simulink model "DCP_model"  (R2015b)
settings: Solver=ode3  StartTime=0.0  StopTime=inf  RelTol=1e-3
values from neighbouring files (symbols this model uses):
  numCars = 3    [Init_script.m]
undefined symbols (not defined in the file or in its folder): cars1, cars2, cars3, const, mat, param
libraries: CarMaker4SL x19, simulink x2
(part 2 of 2)

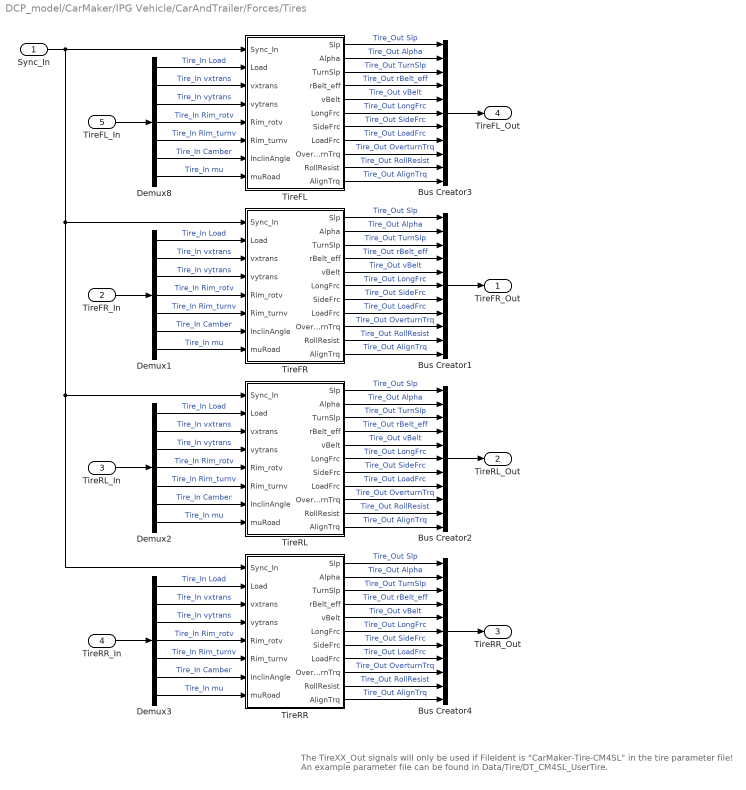
== system DCP_model/CarMaker/IPG Vehicle/CarAndTrailer/Forces/Tires ==
  note: The TireXX_Out signals will only be used if FileIdent is "CarMaker-Tire-CM4SL" in the tire parameter file!
      | An example parameter file can be found in Data/Tire/DT_CM4SL_UserTire.
  Sync_In : Inport
  TireFR_In : Inport  Port=2
  TireRL_In : Inport  Port=3
  TireRR_In : Inport  Port=4
  TireFL_In : Inport  Port=5
  Bus Creator{1..4} (4 alike) : BusCreator  Inputs=11
  Demux{1..3,8} (4 alike) : Demux  Outputs=7
  TireFL : Subsystem
  TireFR : Subsystem
  TireRL : Subsystem
  TireRR : Subsystem
  TireFR_Out : Outport
  TireRL_Out : Outport  Port=2
  TireRR_Out : Outport  Port=3
  TireFL_Out : Outport  Port=4
  wires:
  Sync_In/1 -> TireRR/1(Sync_In), TireRL/1(Sync_In), TireFR/1(Sync_In), TireFL/1(Sync_In)
  Bus Creator4/1 -> TireRR_Out/1
  Bus Creator2/1 -> TireRL_Out/1
  Bus Creator1/1 -> TireFR_Out/1
  Demux3/5 -> TireRR/6(Rim_turnv)  "Tire_In Rim_turnv"
  Demux3/4 -> TireRR/5(Rim_rotv)  "Tire_In Rim_rotv"
  Demux3/1 -> TireRR/2(Load)  "Tire_In Load"
  Demux3/7 -> TireRR/8(muRoad)  "Tire_In mu"
  Demux3/6 -> TireRR/7(InclinAngle)  "Tire_In Camber"
  Demux3/2 -> TireRR/3(vxtrans)  "Tire_In vxtrans"
  Demux3/3 -> TireRR/4(vytrans)  "Tire_In vytrans"
  TireRR/11(AlignTrq) -> Bus Creator4/11  "Tire_Out AlignTrq"
  TireRR/10(RollResist) -> Bus Creator4/10  "Tire_Out RollResist"
  TireRR/9(OverturnTrq) -> Bus Creator4/9  "Tire_Out OverturnTrq"
  TireRR/8(LoadFrc) -> Bus Creator4/8  "Tire_Out LoadFrc"
  TireRR/7(SideFrc) -> Bus Creator4/7  "Tire_Out SideFrc"
  TireRR/6(LongFrc) -> Bus Creator4/6  "Tire_Out LongFrc"
  TireRR/5(vBelt) -> Bus Creator4/5  "Tire_Out vBelt"
  TireRR/4(rBelt_eff) -> Bus Creator4/4  "Tire_Out rBelt_eff"
  TireRR/3(TurnSlp) -> Bus Creator4/3  "Tire_Out TurnSlp"
  TireRR/1(Slp) -> Bus Creator4/1  "Tire_Out Slp"
  TireRR/2(Alpha) -> Bus Creator4/2  "Tire_Out Alpha"
  Demux2/5 -> TireRL/6(Rim_turnv)  "Tire_In Rim_turnv"
  Demux2/4 -> TireRL/5(Rim_rotv)  "Tire_In Rim_rotv"
  Demux2/1 -> TireRL/2(Load)  "Tire_In Load"
  Demux2/7 -> TireRL/8(muRoad)  "Tire_In mu"
  Demux2/6 -> TireRL/7(InclinAngle)  "Tire_In Camber"
  Demux2/2 -> TireRL/3(vxtrans)  "Tire_In vxtrans"
  Demux2/3 -> TireRL/4(vytrans)  "Tire_In vytrans"
  TireRL/11(AlignTrq) -> Bus Creator2/11  "Tire_Out AlignTrq"
  TireRL/10(RollResist) -> Bus Creator2/10  "Tire_Out RollResist"
  TireRL/9(OverturnTrq) -> Bus Creator2/9  "Tire_Out OverturnTrq"
  TireRL/8(LoadFrc) -> Bus Creator2/8  "Tire_Out LoadFrc"
  TireRL/7(SideFrc) -> Bus Creator2/7  "Tire_Out SideFrc"
  TireRL/6(LongFrc) -> Bus Creator2/6  "Tire_Out LongFrc"
  TireRL/5(vBelt) -> Bus Creator2/5  "Tire_Out vBelt"
  TireRL/4(rBelt_eff) -> Bus Creator2/4  "Tire_Out rBelt_eff"
  TireRL/3(TurnSlp) -> Bus Creator2/3  "Tire_Out TurnSlp"
  TireRL/1(Slp) -> Bus Creator2/1  "Tire_Out Slp"
  TireRL/2(Alpha) -> Bus Creator2/2  "Tire_Out Alpha"
  Demux1/5 -> TireFR/6(Rim_turnv)  "Tire_In Rim_turnv"
  Demux1/4 -> TireFR/5(Rim_rotv)  "Tire_In Rim_rotv"
  Demux1/1 -> TireFR/2(Load)  "Tire_In Load"
  Demux1/7 -> TireFR/8(muRoad)  "Tire_In mu"
  Demux1/6 -> TireFR/7(InclinAngle)  "Tire_In Camber"
  Demux1/2 -> TireFR/3(vxtrans)  "Tire_In vxtrans"
  Demux1/3 -> TireFR/4(vytrans)  "Tire_In vytrans"
  TireFR/11(AlignTrq) -> Bus Creator1/11  "Tire_Out AlignTrq"
  TireFR/10(RollResist) -> Bus Creator1/10  "Tire_Out RollResist"
  TireFR/9(OverturnTrq) -> Bus Creator1/9  "Tire_Out OverturnTrq"
  TireFR/8(LoadFrc) -> Bus Creator1/8  "Tire_Out LoadFrc"
  TireFR/7(SideFrc) -> Bus Creator1/7  "Tire_Out SideFrc"
  TireFR/6(LongFrc) -> Bus Creator1/6  "Tire_Out LongFrc"
  TireFR/5(vBelt) -> Bus Creator1/5  "Tire_Out vBelt"
  TireFR/4(rBelt_eff) -> Bus Creator1/4  "Tire_Out rBelt_eff"
  TireFR/3(TurnSlp) -> Bus Creator1/3  "Tire_Out TurnSlp"
  TireFR/1(Slp) -> Bus Creator1/1  "Tire_Out Slp"
  TireFR/2(Alpha) -> Bus Creator1/2  "Tire_Out Alpha"
  Demux8/5 -> TireFL/6(Rim_turnv)  "Tire_In Rim_turnv"
  Demux8/4 -> TireFL/5(Rim_rotv)  "Tire_In Rim_rotv"
  TireFL_In/1 -> Demux8/1
  Demux8/1 -> TireFL/2(Load)  "Tire_In Load"
  Demux8/7 -> TireFL/8(muRoad)  "Tire_In mu"
  Demux8/6 -> TireFL/7(InclinAngle)  "Tire_In Camber"
  Demux8/2 -> TireFL/3(vxtrans)  "Tire_In vxtrans"
  Demux8/3 -> TireFL/4(vytrans)  "Tire_In vytrans"
  TireFL/11(AlignTrq) -> Bus Creator3/11  "Tire_Out AlignTrq"
  TireFL/10(RollResist) -> Bus Creator3/10  "Tire_Out RollResist"
  TireFL/9(OverturnTrq) -> Bus Creator3/9  "Tire_Out OverturnTrq"
  TireFL/8(LoadFrc) -> Bus Creator3/8  "Tire_Out LoadFrc"
  TireFL/7(SideFrc) -> Bus Creator3/7  "Tire_Out SideFrc"
  TireFL/6(LongFrc) -> Bus Creator3/6  "Tire_Out LongFrc"
  TireFL/5(vBelt) -> Bus Creator3/5  "Tire_Out vBelt"
  TireFL/4(rBelt_eff) -> Bus Creator3/4  "Tire_Out rBelt_eff"
  TireFL/3(TurnSlp) -> Bus Creator3/3  "Tire_Out TurnSlp"
  TireFL/1(Slp) -> Bus Creator3/1  "Tire_Out Slp"
  TireFL/2(Alpha) -> Bus Creator3/2  "Tire_Out Alpha"
  Bus Creator3/1 -> TireFL_Out/1
  TireFR_In/1 -> Demux1/1
  TireRL_In/1 -> Demux2/1
  TireRR_In/1 -> Demux3/1

== system DCP_model/CarMaker/IPG Vehicle/CarAndTrailer/Forces/Vehicle Forces ==
  Sync_In : Inport
  Bus Creator1 : BusCreator  Inputs=12
  Bus Creator5 : BusCreator  Inputs=13
  Bus Creator8 : BusCreator  Inputs=16
  Demux : Demux  Outputs=16
  Demux1 : Demux  Outputs=12
  Demux5 : Demux  Outputs=13
  Forces : S-Function  FunctionName=CM_Sfun  Parameters='Forces'  SFunctionDeploymentMode=off  EnableBusSupport=off
  Sync_Out : Outport
  Car.Virtual : Outport  Port=2
  Car.Aero : Outport  Port=3
  Car.Load : Outport  Port=4
  wires:
  Demux/16 -> Bus Creator8/16  "Car Load_3 tz"
  Demux/15 -> Bus Creator8/15  "Car Load_3 ty"
  Demux/14 -> Bus Creator8/14  "Car Load_3 tx"
  Demux/13 -> Bus Creator8/13  "Car Load_3 mass"
  Demux1/12 -> Bus Creator1/12  "Car Virtual Trq_0 z"
  Demux1/11 -> Bus Creator1/11  "Car Virtual Trq_0 y"
  Demux1/10 -> Bus Creator1/10  "Car Virtual Trq_0 x"
  Demux1/9 -> Bus Creator1/9  "Car Virtual Trq_1 z"
  Demux1/8 -> Bus Creator1/8  "Car Virtual Trq_1 y"
  Demux1/7 -> Bus Creator1/7  "Car Virtual Trq_1 x"
  Demux1/6 -> Bus Creator1/6  "Car Virtual Frc_0 z"
  Demux1/5 -> Bus Creator1/5  "Car Virtual Frc_0 y"
  Demux1/4 -> Bus Creator1/4  "Car Virtual Frc_0 x"
  Sync_In/1 -> Forces/1
  Forces/1 -> Sync_Out/1
  Bus Creator5/1 -> Car.Aero/1
  Demux1/1 -> Bus Creator1/1  "Car Virtual Frc_1 x"
  Demux1/2 -> Bus Creator1/2  "Car Virtual Frc_1 y"
  Demux1/3 -> Bus Creator1/3  "Car Virtual Frc_1 z"
  Forces/3 -> Demux5/1
  Forces/2 -> Demux1/1
  Bus Creator1/1 -> Car.Virtual/1
  Bus Creator8/1 -> Car.Load/1
  Demux/1 -> Bus Creator8/1  "Car Load_0 mass"
  Demux/2 -> Bus Creator8/2  "Car Load_0 tx"
  Demux/3 -> Bus Creator8/3  "Car Load_0 ty"
  Demux/4 -> Bus Creator8/4  "Car Load_0 tz"
  Demux/5 -> Bus Creator8/5  "Car Load_1 mass"
  Demux/6 -> Bus Creator8/6  "Car Load_1 tx"
  Demux/7 -> Bus Creator8/7  "Car Load_1 ty"
  Demux/8 -> Bus Creator8/8  "Car Load_1 tz"
  Demux/9 -> Bus Creator8/9  "Car Load_2 mass"
  Demux/10 -> Bus Creator8/10  "Car Load_2 tx"
  Demux/11 -> Bus Creator8/11  "Car Load_2 ty"
  Demux/12 -> Bus Creator8/12  "Car Load_2 tz"
  Forces/4 -> Demux/1
  Demux5/11 -> Bus Creator5/11  "car Aero Trq_1 x"
  Demux5/12 -> Bus Creator5/12  "car Aero Trq_1 y"
  Demux5/13 -> Bus Creator5/13  "car Aero Trq_1 z"
  Demux5/10 -> Bus Creator5/10  "car Aero Frc_1 z"
  Demux5/9 -> Bus Creator5/9  "car Aero Frc_1 y"
  Demux5/8 -> Bus Creator5/8  "car Aero Frc_1 x"
  Demux5/1 -> Bus Creator5/1  "Vehicle sRoadAero"
  Demux5/2 -> Bus Creator5/2  "Vehicle Wind_vel_0 x"
  Demux5/3 -> Bus Creator5/3  "Vehicle Wind_vel_0 y"
  Demux5/4 -> Bus Creator5/4  "Vehicle Wind_vel_0 z"
  Demux5/5 -> Bus Creator5/5  "car Aero vRes_1 x"
  Demux5/6 -> Bus Creator5/6  "car Aero vRes_1 y"
  Demux5/7 -> Bus Creator5/7  "car Aero vRes_1 z"

== system DCP_model/CarMaker/IPG Vehicle/CarAndTrailer/Trailer/CreateBus Car.Hitch.FrcTrq ==
  In1 : Inport
  Bus Creator7 : BusCreator  Inputs=6
  Demux7 : Demux  Outputs=6
  Car.Hitch.FrcTrq : Outport
  wires:
  In1/1 -> Demux7/1
  Bus Creator7/1 -> Car.Hitch.FrcTrq/1
  Demux7/6 -> Bus Creator7/6  "Car Hitch Trq2Car z"
  Demux7/5 -> Bus Creator7/5  "Car Hitch Trq2Car y"
  Demux7/4 -> Bus Creator7/4  "Car Hitch Trq2Car x"
  Demux7/3 -> Bus Creator7/3  "Car Hitch Frc2Car z"
  Demux7/2 -> Bus Creator7/2  "Car Hitch Frc2Car y"
  Demux7/1 -> Bus Creator7/1  "Car Hitch Frc2Car x"

== system DCP_model/CarMaker/IPG Vehicle/CarAndTrailer/Trailer/CreateBus Vhcl.Motion ==
  In1 : Inport
  Demux1 : Demux  Outputs=16
  Mux1 : Mux  Inputs=16
  Out1 : Outport
  wires:
  Demux1/1 -> Mux1/1  "Vhcl v"
  Demux1/2 -> Mux1/2  "Vhcl Distance"
  Demux1/3 -> Mux1/3  "Vhcl sRoad"
  Demux1/4 -> Mux1/4  "Vhcl sRoadAero"
  Demux1/5 -> Mux1/5  "Vhcl Hitch_Pos x"
  Demux1/6 -> Mux1/6  "Vhcl Hitch_Pos y"
  Demux1/7 -> Mux1/7  "Vhcl Hitch_Pos z"
  Demux1/8 -> Mux1/8  "Vhcl Roll"
  Demux1/9 -> Mux1/9  "Vhcl RollVel"
  Demux1/10 -> Mux1/10  "Vhcl RollAcc"
  Demux1/11 -> Mux1/11  "Vhcl Pitch"
  Demux1/12 -> Mux1/12  "Vhcl PitchVel"
  Demux1/13 -> Mux1/13  "Vhcl PitchAcc"
  Demux1/14 -> Mux1/14  "Vhcl Yaw"
  Demux1/15 -> Mux1/15  "Vhcl YawRate"
  Demux1/16 -> Mux1/16  "Vhcl YawAcc"
  In1/1 -> Demux1/1
  Mux1/1 -> Out1/1

== system DCP_model/CarMaker/IPG Vehicle/CarAndTrailer/Trailer/CreateBus Vhcl.PoI ==
  In1 : Inport
  Bus Creator3 : BusCreator  Inputs=18
  Demux3 : Demux  Outputs=18
  Out1 : Outport
  wires:
  Demux3/18 -> Bus Creator3/18  "Vhcl PoI_GCS Elev"
  Demux3/17 -> Bus Creator3/17  "Vhcl PoI_GCS Lat"
  Demux3/16 -> Bus Creator3/16  "Vhcl PoI_GCS Long"
  Demux3/15 -> Bus Creator3/15  "Vhcl PoI_Acc_1 z"
  Demux3/14 -> Bus Creator3/14  "Vhcl PoI_Acc_1 y"
  Demux3/13 -> Bus Creator3/13  "Vhcl PoI_Acc_1 x"
  Demux3/12 -> Bus Creator3/12  "Vhcl PoI_Vel_1 z"
  Demux3/11 -> Bus Creator3/11  "Vhcl PoI_Vel_1 y"
  Demux3/10 -> Bus Creator3/10  "Vhcl PoI_Vel_1 x"
  Demux3/9 -> Bus Creator3/9  "Vhcl PoI_Acc z"
  Demux3/8 -> Bus Creator3/8  "Vhcl PoI_Acc y"
  Demux3/7 -> Bus Creator3/7  "Vhcl PoI_Acc x"
  Demux3/6 -> Bus Creator3/6  "Vhcl PoI_Vel z"
  Demux3/5 -> Bus Creator3/5  "Vhcl PoI_Vel y"
  Demux3/4 -> Bus Creator3/4  "Vhcl PoI_Vel x"
  Demux3/3 -> Bus Creator3/3  "Vhcl PoI_Pos z"
  Demux3/2 -> Bus Creator3/2  "Vhcl PoI_Pos y"
  In1/1 -> Demux3/1
  Bus Creator3/1 -> Out1/1
  Demux3/1 -> Bus Creator3/1  "Vhcl PoI_Pos x"

== system DCP_model/CarMaker/IPG Vehicle/CarAndTrailer/Trailer/CreateBus Vhcl.Steering ==
  In1 : Inport
  Bus Creator3 : BusCreator  Inputs=4
  Demux : Demux
  Out1 : Outport
  wires:
  Bus Creator3/1 -> Out1/1
  Demux/1 -> Bus Creator3/1  "Vhcl Steering Ang"
  Demux/3 -> Bus Creator3/3  "Vhcl Steering AngAcc"
  Demux/2 -> Bus Creator3/2  "Vhcl Steering AngVel"
  Demux/4 -> Bus Creator3/4  "Vhcl Steering Trq"
  In1/1 -> Demux/1

== system DCP_model/CarMaker/IPG Vehicle/CarAndTrailer/Trailer/CreateBus Vhcl.Wheel.FL ==
  In1 : Inport
  Bus Creator3 : BusCreator  Inputs=14
  Demux3 : Demux  Outputs=14
  Out1 : Outport
  wires:
  Demux3/14 -> Bus Creator3/14  "Vhcl Wheel FL Trq_WhlBearing"
  Demux3/13 -> Bus Creator3/13  "Vhcl Wheel FL Trq_T2W"
  Demux3/12 -> Bus Creator3/12  "Vhcl Wheel FL SideSlip"
  Demux3/11 -> Bus Creator3/11  "Vhcl Wheel FL LongSlip"
  Demux3/10 -> Bus Creator3/10  "Vhcl Wheel FL vBelt"
  Demux3/9 -> Bus Creator3/9  "Vhcl Wheel FL Fz"
  Demux3/8 -> Bus Creator3/8  "Vhcl Wheel FL Fy"
  Demux3/7 -> Bus Creator3/7  "Vhcl Wheel FL Fx"
  Demux3/6 -> Bus Creator3/6  "Vhcl Wheel FL r_zxy z"
  Demux3/5 -> Bus Creator3/5  "Vhcl Wheel FL r_zxy y"
  Demux3/4 -> Bus Creator3/4  "Vhcl Wheel FL r_zxy x"
  Demux3/3 -> Bus Creator3/3  "Vhcl Wheel FL t z"
  Demux3/2 -> Bus Creator3/2  "Vhcl Wheel FL t y"
  In1/1 -> Demux3/1
  Bus Creator3/1 -> Out1/1
  Demux3/1 -> Bus Creator3/1  "Vhcl Wheel FL t x"

== system DCP_model/CarMaker/IPG Vehicle/CarAndTrailer/Trailer/CreateBus Vhcl.Wheel.FR ==
  In1 : Inport
  Bus Creator3 : BusCreator  Inputs=14
  Demux3 : Demux  Outputs=14
  Out1 : Outport
  wires:
  Demux3/14 -> Bus Creator3/14  "Vhcl Wheel FR Trq_WhlBearing"
  Demux3/13 -> Bus Creator3/13  "Vhcl Wheel FR Trq_T2W"
  Demux3/12 -> Bus Creator3/12  "Vhcl Wheel FR SideSlip"
  Demux3/11 -> Bus Creator3/11  "Vhcl Wheel FR LongSlip"
  Demux3/10 -> Bus Creator3/10  "Vhcl Wheel FR vBelt"
  Demux3/9 -> Bus Creator3/9  "Vhcl Wheel FR Fz"
  Demux3/8 -> Bus Creator3/8  "Vhcl Wheel FR Fy"
  Demux3/7 -> Bus Creator3/7  "Vhcl Wheel FR Fx"
  Demux3/6 -> Bus Creator3/6  "Vhcl Wheel FR r_zxy z"
  Demux3/5 -> Bus Creator3/5  "Vhcl Wheel FR r_zxy y"
  Demux3/4 -> Bus Creator3/4  "Vhcl Wheel FR r_zxy x"
  Demux3/3 -> Bus Creator3/3  "Vhcl Wheel FR t z"
  Demux3/2 -> Bus Creator3/2  "Vhcl Wheel FR t y"
  In1/1 -> Demux3/1
  Bus Creator3/1 -> Out1/1
  Demux3/1 -> Bus Creator3/1  "Vhcl Wheel FR t x"

== system DCP_model/CarMaker/IPG Vehicle/CarAndTrailer/Trailer/CreateBus Vhcl.Wheel.RL ==
  In1 : Inport
  Bus Creator3 : BusCreator  Inputs=14
  Demux3 : Demux  Outputs=14
  Out1 : Outport
  wires:
  Demux3/14 -> Bus Creator3/14  "Vhcl Wheel RL Trq_WhlBearing"
  Demux3/13 -> Bus Creator3/13  "Vhcl Wheel RL Trq_T2W"
  Demux3/12 -> Bus Creator3/12  "Vhcl Wheel RL SideSlip"
  Demux3/11 -> Bus Creator3/11  "Vhcl Wheel RL LongSlip"
  Demux3/10 -> Bus Creator3/10  "Vhcl Wheel RL vBelt"
  Demux3/9 -> Bus Creator3/9  "Vhcl Wheel RL Fz"
  Demux3/8 -> Bus Creator3/8  "Vhcl Wheel RL Fy"
  Demux3/7 -> Bus Creator3/7  "Vhcl Wheel RL Fx"
  Demux3/6 -> Bus Creator3/6  "Vhcl Wheel RL r_zxy z"
  Demux3/5 -> Bus Creator3/5  "Vhcl Wheel RL r_zxy y"
  Demux3/4 -> Bus Creator3/4  "Vhcl Wheel RL r_zxy x"
  Demux3/3 -> Bus Creator3/3  "Vhcl Wheel RL t z"
  Demux3/2 -> Bus Creator3/2  "Vhcl Wheel RL t y"
  In1/1 -> Demux3/1
  Bus Creator3/1 -> Out1/1
  Demux3/1 -> Bus Creator3/1  "Vhcl Wheel RL t x"

== system DCP_model/CarMaker/IPG Vehicle/CarAndTrailer/Trailer/CreateBus Vhcl.Wheel.RR ==
  In1 : Inport
  Bus Creator3 : BusCreator  Inputs=14
  Demux3 : Demux  Outputs=14
  Out1 : Outport
  wires:
  Demux3/14 -> Bus Creator3/14  "Vhcl Wheel RR Trq_WhlBearing"
  Demux3/13 -> Bus Creator3/13  "Vhcl Wheel RR Trq_T2W"
  Demux3/12 -> Bus Creator3/12  "Vhcl Wheel RR SideSlip"
  Demux3/11 -> Bus Creator3/11  "Vhcl Wheel RR LongSlip"
  Demux3/10 -> Bus Creator3/10  "Vhcl Wheel RR vBelt"
  Demux3/9 -> Bus Creator3/9  "Vhcl Wheel RR Fz"
  Demux3/8 -> Bus Creator3/8  "Vhcl Wheel RR Fy"
  Demux3/7 -> Bus Creator3/7  "Vhcl Wheel RR Fx"
  Demux3/6 -> Bus Creator3/6  "Vhcl Wheel RR r_zxy z"
  Demux3/5 -> Bus Creator3/5  "Vhcl Wheel RR r_zxy y"
  Demux3/4 -> Bus Creator3/4  "Vhcl Wheel RR r_zxy x"
  Demux3/3 -> Bus Creator3/3  "Vhcl Wheel RR t z"
  Demux3/2 -> Bus Creator3/2  "Vhcl Wheel RR t y"
  In1/1 -> Demux3/1
  Bus Creator3/1 -> Out1/1
  Demux3/1 -> Bus Creator3/1  "Vhcl Wheel RR t x"

== system DCP_model/CarMaker/VehicleControl/AccelCtrl1/PI-Controller/Integrator ==
  I-Part : Inport
  AxCtrl On : Inport  Port=2
  Init I-part : Inport  Port=3
  Add1 : Sum  SaturateOnIntegerOverflow=on  OutDataTypeStr=Inherit: Same as first input
  Memory : Memory
  Saturation : Saturate  UpperLimit=1  LowerLimit=-1
  Switch Ax Init I-Part : Switch  Threshold=1  SaturateOnIntegerOverflow=on
  "I-part tot " : Outport
  wires:
  Init I-part/1 -> Switch Ax Init I-Part/3
  Memory/1 -> Switch Ax Init I-Part/1
  AxCtrl On/1 -> Switch Ax Init I-Part/2
  I-Part/1 -> Add1/1
  Add1/1 -> "I-part tot "/1, Saturation/1
  Switch Ax Init I-Part/1 -> Add1/2
  Saturation/1 -> Memory/1

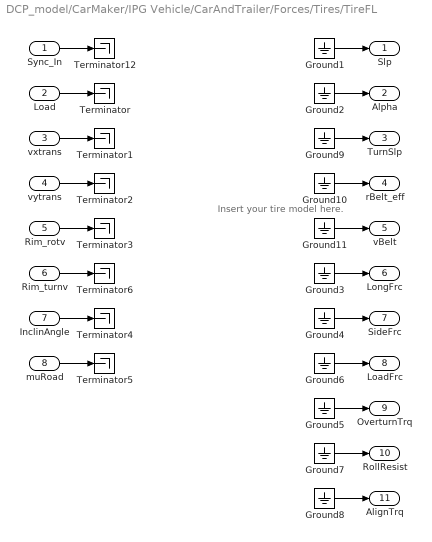
== system DCP_model/CarMaker/IPG Vehicle/CarAndTrailer/Forces/Tires/TireFL ==
  note: Insert your tire model here.
  Sync_In : Inport
  Load : Inport  Port=2
  vxtrans : Inport  Port=3
  vytrans : Inport  Port=4
  Rim_rotv : Inport  Port=5
  Rim_turnv : Inport  Port=6
  InclinAngle : Inport  Port=7
  muRoad : Inport  Port=8
  Ground{1..11} (11 alike) : Ground
  Terminator{,1..6,12} (8 alike) : Terminator
  Slp : Outport
  Alpha : Outport  Port=2
  TurnSlp : Outport  Port=3
  rBelt_eff : Outport  Port=4
  vBelt : Outport  Port=5
  LongFrc : Outport  Port=6
  SideFrc : Outport  Port=7
  LoadFrc : Outport  Port=8
  OverturnTrq : Outport  Port=9
  RollResist : Outport  Port=10
  AlignTrq : Outport  Port=11
  wires:
  Ground11/1 -> vBelt/1
  Ground10/1 -> rBelt_eff/1
  Ground9/1 -> TurnSlp/1
  Rim_turnv/1 -> Terminator6/1
  Sync_In/1 -> Terminator12/1
  Ground2/1 -> Alpha/1
  Ground3/1 -> LongFrc/1
  Ground4/1 -> SideFrc/1
  Ground5/1 -> OverturnTrq/1
  vxtrans/1 -> Terminator1/1
  vytrans/1 -> Terminator2/1
  Rim_rotv/1 -> Terminator3/1
  InclinAngle/1 -> Terminator4/1
  muRoad/1 -> Terminator5/1
  Load/1 -> Terminator/1
  Ground1/1 -> Slp/1
  Ground6/1 -> LoadFrc/1
  Ground7/1 -> RollResist/1
  Ground8/1 -> AlignTrq/1

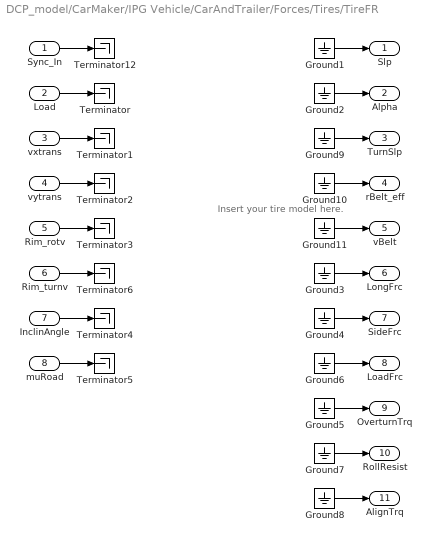
== system DCP_model/CarMaker/IPG Vehicle/CarAndTrailer/Forces/Tires/TireFR ==
  note: Insert your tire model here.
  Sync_In : Inport
  Load : Inport  Port=2
  vxtrans : Inport  Port=3
  vytrans : Inport  Port=4
  Rim_rotv : Inport  Port=5
  Rim_turnv : Inport  Port=6
  InclinAngle : Inport  Port=7
  muRoad : Inport  Port=8
  Ground{1..11} (11 alike) : Ground
  Terminator{,1..6,12} (8 alike) : Terminator
  Slp : Outport
  Alpha : Outport  Port=2
  TurnSlp : Outport  Port=3
  rBelt_eff : Outport  Port=4
  vBelt : Outport  Port=5
  LongFrc : Outport  Port=6
  SideFrc : Outport  Port=7
  LoadFrc : Outport  Port=8
  OverturnTrq : Outport  Port=9
  RollResist : Outport  Port=10
  AlignTrq : Outport  Port=11
  wires:
  Ground11/1 -> vBelt/1
  Ground10/1 -> rBelt_eff/1
  Ground9/1 -> TurnSlp/1
  Rim_turnv/1 -> Terminator6/1
  Sync_In/1 -> Terminator12/1
  Ground2/1 -> Alpha/1
  Ground3/1 -> LongFrc/1
  Ground4/1 -> SideFrc/1
  Ground5/1 -> OverturnTrq/1
  vxtrans/1 -> Terminator1/1
  vytrans/1 -> Terminator2/1
  Rim_rotv/1 -> Terminator3/1
  InclinAngle/1 -> Terminator4/1
  muRoad/1 -> Terminator5/1
  Load/1 -> Terminator/1
  Ground1/1 -> Slp/1
  Ground6/1 -> LoadFrc/1
  Ground7/1 -> RollResist/1
  Ground8/1 -> AlignTrq/1

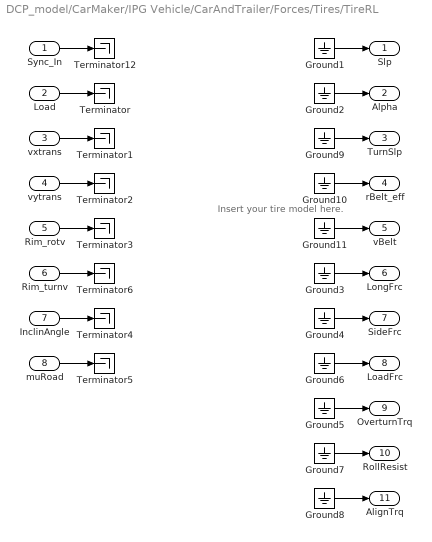
== system DCP_model/CarMaker/IPG Vehicle/CarAndTrailer/Forces/Tires/TireRL ==
  note: Insert your tire model here.
  Sync_In : Inport
  Load : Inport  Port=2
  vxtrans : Inport  Port=3
  vytrans : Inport  Port=4
  Rim_rotv : Inport  Port=5
  Rim_turnv : Inport  Port=6
  InclinAngle : Inport  Port=7
  muRoad : Inport  Port=8
  Ground{1..11} (11 alike) : Ground
  Terminator{,1..6,12} (8 alike) : Terminator
  Slp : Outport
  Alpha : Outport  Port=2
  TurnSlp : Outport  Port=3
  rBelt_eff : Outport  Port=4
  vBelt : Outport  Port=5
  LongFrc : Outport  Port=6
  SideFrc : Outport  Port=7
  LoadFrc : Outport  Port=8
  OverturnTrq : Outport  Port=9
  RollResist : Outport  Port=10
  AlignTrq : Outport  Port=11
  wires:
  Ground11/1 -> vBelt/1
  Ground10/1 -> rBelt_eff/1
  Ground9/1 -> TurnSlp/1
  Rim_turnv/1 -> Terminator6/1
  Sync_In/1 -> Terminator12/1
  Ground2/1 -> Alpha/1
  Ground3/1 -> LongFrc/1
  Ground4/1 -> SideFrc/1
  Ground5/1 -> OverturnTrq/1
  vxtrans/1 -> Terminator1/1
  vytrans/1 -> Terminator2/1
  Rim_rotv/1 -> Terminator3/1
  InclinAngle/1 -> Terminator4/1
  muRoad/1 -> Terminator5/1
  Load/1 -> Terminator/1
  Ground1/1 -> Slp/1
  Ground6/1 -> LoadFrc/1
  Ground7/1 -> RollResist/1
  Ground8/1 -> AlignTrq/1

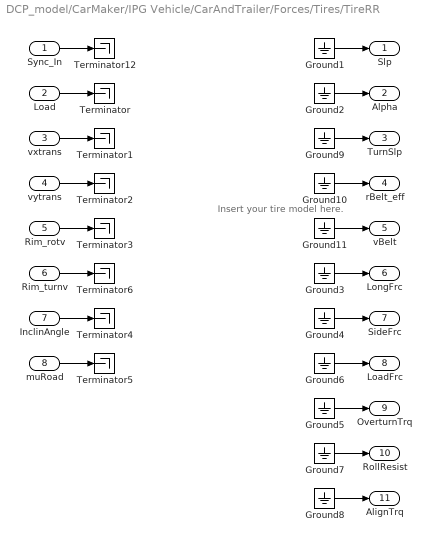
== system DCP_model/CarMaker/IPG Vehicle/CarAndTrailer/Forces/Tires/TireRR ==
  note: Insert your tire model here.
  Sync_In : Inport
  Load : Inport  Port=2
  vxtrans : Inport  Port=3
  vytrans : Inport  Port=4
  Rim_rotv : Inport  Port=5
  Rim_turnv : Inport  Port=6
  InclinAngle : Inport  Port=7
  muRoad : Inport  Port=8
  Ground{1..11} (11 alike) : Ground
  Terminator{,1..6,12} (8 alike) : Terminator
  Slp : Outport
  Alpha : Outport  Port=2
  TurnSlp : Outport  Port=3
  rBelt_eff : Outport  Port=4
  vBelt : Outport  Port=5
  LongFrc : Outport  Port=6
  SideFrc : Outport  Port=7
  LoadFrc : Outport  Port=8
  OverturnTrq : Outport  Port=9
  RollResist : Outport  Port=10
  AlignTrq : Outport  Port=11
  wires:
  Ground11/1 -> vBelt/1
  Ground10/1 -> rBelt_eff/1
  Ground9/1 -> TurnSlp/1
  Rim_turnv/1 -> Terminator6/1
  Sync_In/1 -> Terminator12/1
  Ground2/1 -> Alpha/1
  Ground3/1 -> LongFrc/1
  Ground4/1 -> SideFrc/1
  Ground5/1 -> OverturnTrq/1
  vxtrans/1 -> Terminator1/1
  vytrans/1 -> Terminator2/1
  Rim_rotv/1 -> Terminator3/1
  InclinAngle/1 -> Terminator4/1
  muRoad/1 -> Terminator5/1
  Load/1 -> Terminator/1
  Ground1/1 -> Slp/1
  Ground6/1 -> LoadFrc/1
  Ground7/1 -> RollResist/1
  Ground8/1 -> AlignTrq/1

== matlab function DCP_model/CarMaker/VehicleControl/Subsystem/MATLAB Function1 ==
  data: longAcc output; param parameter; const parameter; mat parameter; cars1 parameter; cars2 parameter; cars3 parameter; numCars parameter; dist2Int input; uk input; upk input; time input; velocity input; uk1 output; upk1 output; exflag output
function [longAcc,uk1,upk1,exflag]   = MPC (param,const,mat,cars1,cars2,cars3,numCars,dist2Int,uk,upk,time,velocity)  %#codegen

coder.extrinsic('quadprog');
exflag = zeros(1,1,'double');

% system Matrices
A = mat.A; 
B = mat.B; 
C = mat.C'; 
Q = mat.Qv;

% parameter data
contR = param.contrRadius;
critZ = param.critZone;
w = [param.weights];
ds = param.sampling;
tdiff = param.timediff;


refVel = zeros(1,3);
meanVel = zeros(1,3);

refVel(1) = cars1.refVel;
refVel(2) = cars2.refVel;
refVel(3) = cars3.refVel; 

meanVel(1) = cars1.meanVel;
meanVel(2) = cars2.meanVel;
meanVel(3) = cars3.meanVel;


xk = zeros(2,3);

xk(:,1) = [time; 1/velocity(1)];
xk(:,2) = [time; 1/velocity(2)];
xk(:,3) = [time; 1/velocity(3)];

longAcc = zeros(3,1);
uk1 = zeros(3,1);
upk1 = zeros(3,1);
No = 2*contR + critZ; % maximum prediction horizon

% Constraints
amax = const.amax; amin = const.amin ;
vmax = const.vmax ; vmin = const.vmin ;

% N = 2*contR + critZ + (car(j).dist2Int - contR) = contR+critZ+car(j).dist2Int

% Prediction horizon for each cars
N = contR+critZ+dist2Int;
N(N < 0 | N > No) = 0; % The car have to be inside the control horizon

HM11 = zeros(270,270);
HM21 = zeros(135,135);
HM31 = zeros(135,135);

Hm1 = zeros(4*135,4*135);
f1 = zeros(4*135,1);

Ha1 = zeros(2*135,2*135);
Hi1 = zeros(2*135,2*135);

Hi11 = zeros(135-1, 135);
Hi21 = zeros(135-1, 135);

Aeq1 = zeros(3*135+1,4*135);
beq1 = zeros(3*135+1,1);

Ain1 = zeros(4*135,4*135);
bin1 = zeros(4*135,1);
  

coder.varsize('HM11', [270 270], [1 1]);
coder.varsize('HM21');
coder.varsize('HM31');
coder.varsize('Hm1');
coder.varsize('f1');
coder.varsize('Ha1');
coder.varsize('Hi1');
coder.varsize('Hi11');
coder.varsize('Hi21');
coder.varsize('Aeq1');
coder.varsize('beq1');
coder.varsize('Ain1');
coder.varsize('bin1');


% eye zeros and ones also needed to be predifined
Eye = eye(2*135);
coder.varsize('Eye');

Zeros = zeros(4*135,4*135);
coder.varsize('Zeros');

Ones = ones(4*135,4*135);
coder.varsize('Ones');

Neq = [0 0 0];

coder.varsize('Hm',[1620 1620]);

% struct containing all matices for one car
c = [struct('HM1',HM11,'HM2',HM21,'HM3',HM31,'Hm',Hm1,'f',f1,'Ha',Ha1,...
    'Hi',Hi1,'Hi1',Hi11,'Hi2',Hi21,'Aeq',Aeq1,'beq',beq1,'Ain',Ain1,'bin',bin1),...
     struct('HM1',HM11,'HM2',HM21,'HM3',HM31,'Hm',Hm1,'f',f1,'Ha',Ha1,...
    'Hi',Hi1,'Hi1',Hi11,'Hi2',Hi21,'Aeq',Aeq1,'beq',beq1,'Ain',Ain1,'bin',bin1),...
     struct('HM1',HM11,'HM2',HM21,'HM3',HM31,'Hm',Hm1,'f',f1,'Ha',Ha1,...
    'Hi',Hi1,'Hi1',Hi11,'Hi2',Hi21,'Aeq',Aeq1,'beq',beq1,'Ain',Ain1,'bin',bin1)];

for j=1:numCars
       
    % When a car is inside the control region the car
    % will be controlled of by the MPC. The horizon is limited to the exit
    % of the control region.
    if dist2Int(j) <= contR &&  dist2Int(j) > -(contR+critZ)
        
% Hessian Matrix and f vector        

        c(j).HM1(1:2*N(j),1:2*N(j)) = kron(Eye(1:N(j),1:N(j)),2*Q*w(1)*meanVel(j)^3);  % Part J1 opt fcn 
        c(j).HM2(1:N(j),1:N(j)) = kron(Eye(1:N(j),1:N(j)),2*w(2)*meanVel(j)^5);    % Part J2 A opt fcn
        c(j).HM3(1:N(j),1:N(j)) = kron(Eye(1:N(j),1:N(j)),2*w(3)*meanVel(j)^7);    % Part J2 B opt fcn

        c(j).Hm(1:4*N(j),1:4*N(j)) = [c(j).HM1(1:2*N(j),1:2*N(j)) Zeros(1:2*N(j),1:2*N(j))
                   Zeros(1:N(j),1:2*N(j)) c(j).HM2(1:N(j),1:N(j)) Zeros(1:N(j),1:N(j))
                   Zeros(1:N(j),1:3*N(j)) c(j).HM3(1:N(j),1:N(j))];
        
        c(j).f(1:4*N(j),1) = [kron(Ones(1,1:N(j)),-2*1/refVel(j)*w(1)*meanVel(j)^3*C') Zeros(1,1:2*N(j))]'; 
        
% Equality contraints
        
        % help matrices for c.Aeq
        c(j).Ha(1:2*N(j),1:2*N(j)) = [Zeros(1:2,1:2*N(j)); kron(Eye(1:(N(j)-1),1:(N(j)-1)),[1 1;0 1]) Zeros(1:(N(j)-1)*2,1:2)];
        c(j).Hi(1:2*N(j),1:2*N(j)) = Eye(1:N(j)*2,1:N(j)*2);
        c(j).Hi1(1:N(j)-1,1:N(j)) = [Eye(1:N(j)-1,1:N(j)-1) Zeros(1:(N(j)-1),1)];
        c(j).Hi2(1:N(j)-1,1:N(j)) = [Zeros(1:(N(j)-1),1) Eye(1:N(j)-1,1:N(j)-1)];
              
        Neq(j) = 3*N(j) + 1; 
        c(j).Aeq(1:(3*N(j)+1),1:4*N(j)) = ([c(j).Ha(1:2*N(j),1:2*N(j))-c(j).Hi(1:2*N(j),1:2*N(j)) kron(Eye(1:N(j),1:N(j)),B) Zeros(1:2*N(j),1:N(j))    % x+ = Ax + Bu
            Zeros(1:N(j)-1,1:2*N(j)) (c(j).Hi2(1:N(j)-1,1:N(j))-c(j).Hi1(1:N(j)-1,1:N(j)))/ds c(j).Hi1(1:N(j)-1,1:N(j)) % ]);     % u'(k) = (u(k+1) - u(k))/ds
            Zeros(1,1:2*N(j)) 1 Zeros(1,1:2*N(j)-1)         % u(k) = u(k-1) 
            Zeros(1,1:3*N(j)) 1 Zeros(1,1:N(j)-1)]);      % up(k) = up(k-1)


        c(j).beq(1:3*N(j)+1,1) = [-A*xk(:,j) % -A*x(0)
            Zeros(1:N(j)*3-3,1)  
            uk(j)    % u(k) = u(k-1)
            upk(j)]; % up(k) = up(k-1)
                 
        
% Inequality Constraints
        c(j).Ain(1:4*N(j),1:4*N(j)) = [kron(Eye(1:N(j),1:N(j)),C') Zeros(1:N(j),1:2*N(j))  % C*x <= 1/vmin       -> (1)
            kron(Eye(1:N(j),1:N(j)),-C') Zeros(1:N(j),1:2*N(j))                    % -C*x <= -1/vmax     -> (2)
            kron(Eye(1:N(j),1:N(j)),-3*amax/velocity(j)^2*C') -Eye(1:N(j),1:N(j)) Zeros(1:N(j),1:N(j)) % -> (3)
            kron(Eye(1:N(j),1:N(j)),3*amin/velocity(j)^2*C') Eye(1:N(j),1:N(j)) Zeros(1:N(j),1:N(j))]; % -> (4)

        
         c(j).bin(1:4*N(j),1) = [Ones(1:N(j),1).*1/vmin  % (1)
            Ones(1:N(j),1).*(-1/vmax)                    % (2)
            Ones(1:N(j),1).*(-2*amax/velocity(j)^3)      % (3)
            Ones(1:N(j),1).*(2*amin/velocity(j)^3)];     % (4)
        
    else
        c(j).Hm = []; c(j).f = [];
        c(j).Aeq = []; c(j).beq = [];
        c(j).Ain = []; c(j).bin = [];
    end
end



% Cronologic crossing order Car 1-> Car 2 -> Car 3
% -------------------

% index for cars inside control region
ind = find(dist2Int< contR &  dist2Int > -(contR+critZ));
leni = length(ind);

Aeq = blkdiag(c(1).Aeq(1:Neq(1),1:4*N(1)),c(2).Aeq(1:Neq(2),1:4*N(2)),c(3).Aeq(1:Neq(3),1:4*N(3)));
coder.varsize('Aeq',[3*4*135+2, 3*4*135+2]);
n = 0;
if  leni >= 2 % if 2 or more cars is in the control region
 
  
    for j=1: length(ind)-1
        leave = (dist2Int(ind(j))+critZ); % index [m] for first car to leave
        enter = (dist2Int(ind(j+1))); % index [m] for next car to enter
        
        
        if min(leave,enter) >= 1
            n = n+1;
            Aeq = blkdiag(Aeq,0);            
            Aeq(end,2*leave-1 + 4*sum(N(1:(ind(j)-1)))) = -1;
            Aeq(end,2*enter-1 + 4*sum(N(1:(ind(j+1)-1)))) = 1;
            Aeq(end,4*sum(N)+n) = -1;
            
        end
    end
end

H4 = kron(Eye(1:n,1:n),2*w(4));
f4 = kron(Ones(1:n,1),-2*w(4)*tdiff);

beq4 = Zeros(1:n,1);
Ain4 = -Eye(1:n,1:n);
bin4 = Zeros(1:n,1);

coder.varsize('H4','f4','Aeq4','beq4','Ain4','bin4')
% Combined Hessian Matrix and f vector
% ----------------------
Hm = blkdiag(c(1).Hm(1:4*N(1),1:4*N(1)),c(2).Hm(1:4*N(2),1:4*N(2)),c(3).Hm(1:4*N(3),1:4*N(3)),H4);
f = vertcat(c(1).f(1:4*N(1),1),c(2).f(1:4*N(2),1),c(3).f(1:4*N(3),1),f4);

% Equality Constraints Ain*x == bin
% ----------------------

% Aeq = blkdiag(c(1).Aeq(1:Neq(1),1:4*N(1)),c(2).Aeq(1:Neq(2),1:4*N(2)),c(3).Aeq(1:Neq(3),1:4*N(3)),Aeq4);
beq = vertcat(c(1).beq(1:Neq(1),1),c(2).beq(1:Neq(2),1),c(3).beq(1:Neq(3),1),beq4);


% In-Equality Constraints Ain*x <= bin
% ----------------------
Ain = blkdiag(c(1).Ain(1:4*N(1),1:4*N(1)),c(2).Ain(1:4*N(2),1:4*N(2)),c(3).Ain(1:4*N(3),1:4*N(3)),Ain4);

bin = vertcat(c(1).bin(1:4*N(1),1),c(2).bin(1:4*N(2),1),c(3).bin(1:4*N(3),1),bin4);


% Configuration quadprog
% ----------------------
%coder.extrinsic('optimset');
%options = optimset('Algorithm','interior-point-convex','Display','off');


% If any car is within the control region the MPC will optimize the path
% for all cars within the controlling region.
if ~isempty(Hm)
    
    x = zeros(size(Hm,2),1);
    
    
    % tic;
    [x,~,exflag] = quadprog(Hm,f,Ain,bin,Aeq,beq,[],[],[]); %,options);
    % time = toc;
    
%     if exflag == -2
%         disp('Error: exflag == 2 ');
%     end
    
    for j=1:numCars
        
        prev = 4*sum(N(1:j-1));
        
        if N(j) > 2
            longAcc(j) = -x(2*N(j)+2 + prev)/ x(4 + prev)^3;
            uk1(j) = x(2*N(j)+2 + prev);
            upk1(j) = x(3*N(j)+2 + prev);
        else
            longAcc(j) = 0; 
            uk1(j) = 0;
            upk1(j) = 0;
        end
        
    end
    
else
    for j=1:numCars
        longAcc(j) = 0;
        uk1(j) = 0;
        upk1(j) = 0;
    end
end

== matlab function DCP_model/CarMaker/VehicleControl/Subsystem/MATLAB Function2 ==
  data: longAcc output; param parameter; const parameter; mat parameter; cars1 parameter; cars2 parameter; cars3 parameter; dist2Int input; ax input; time input; vx input; exflag output
function [longAcc,exflag]   = MPC (param,const,mat,cars1,cars2,cars3,dist2Int,ax,time,vx)  %#codegen

exflag = zeros(1,1,'double');

% system Matrices
A = mat.A; 
B = mat.B; 
C = mat.C'; 
Qv = mat.Qv;
Qt = mat.Qt;


% parameter data
contR = 60; % Controlradius in meters
critZ = 10; % Critical Zone in meters
ds = 1;     % meters between each sample
numCars = 3;

w = param.weights;
tdiff = param.timediff; % time gap between car 1 leaves and car 2 enters the intersection 
T = param.T; % sampling time
% Constraints
amax = const.amax; amin = const.amin ;
vmax = const.vmax ; vmin = const.vmin ;


refVel = [cars1.refVel, cars2.refVel, cars3.refVel]; 
meanVel = [cars1.meanVel, cars2.meanVel, cars3.meanVel];


% current states for all cars
xk = [time, time, time;
     1/vx(1), 1/vx(2), 1/vx(3)];

uk = -xk(2,:).^3.*ax';
 
  
  
longAcc = zeros(3,1);
No = 2*contR + critZ; % maximum prediction horizon



% N = 2*contR + critZ + (car(j).dist2Int - contR) = contR+critZ+car(j).dist2Int

% Prediction horizon for each cars
N = contR+critZ+dist2Int;
N(N < 0 | N > No) = 0; % The car have to be inside the control horizon

% % % eye zeros and ones also needed to be predifined
Eye = eye(2*135);
% coder.varsize('Eye');
% % 
Zeros = zeros(1170,4*135);
% coder.varsize('Zeros');
% % 
Ones = ones(4*135,4*135);
% coder.varsize('Ones');

Hm = [];
f = [];
Aeq = [];
beq = [];
Ain = [];
bin = [];

coder.varsize('Hm',[1562, 1562],[1,1]);
coder.varsize('f',[1562,1],[1,0]);
coder.varsize('Aeq',[1170,1562],[1,1]);
coder.varsize('beq',[1170,1],[1,0]);
coder.varsize('Ain',[1566,1562],[1,1]);
coder.varsize('bin',[1566,1],[1,0]);
% 
for j=1:numCars
       
    % When a car is inside the control region the car
    % will be controlled of by the MPC. The horizon is limited to the exit
    % of the control region.
    if dist2Int(j) <= contR &&  dist2Int(j) > -(contR+critZ)
        
% % Hessian Matrix and f vector        
    Hj1 = kron(Eye(1:N(j),1:N(j)),2*Qv*w(1)*meanVel(j)^3) + kron(Eye(1:N(j),1:N(j)),Qt*0.00001);
    Hj2 = kron(Eye(1:N(j),1:N(j)),2*w(2)*meanVel(j)^5);
    Hj3 = kron(Eye(1:N(j),1:N(j)),2*w(3)*meanVel(j)^7);
    
    Hm = blkdiag(Hm,Hj1,Hj2,Hj3);
    f = [f; kron(Ones(1:N(j),1),-2*1/refVel(j)*w(1)*meanVel(j)^3*C); Zeros(1:2*N(j),1)];

% % Equality contraints
         
    Ha = [Zeros(1:2,1:2*N(j)); 
          kron(Eye(1:N(j)-1,1:N(j)-1),A) Zeros(1:(N(j)-1)*2,1:2)]; % multiply x(k) with A
    Huk = [Zeros(1,1:N(j));
           Eye(1:N(j)-1,1:N(j)-1) Zeros(1:N(j)-1,1)];     % select all u(k)
    Hukp1 = Eye(1:N(j),1:N(j)); % select all u(k+1)

    
    Aeq_car = [Ha-Eye(1:2*N(j),1:2*N(j)), kron(Eye(1:N(j),1:N(j)),B), Zeros(1:2*N(j),1:N(j)); % A*x(k)-I(2)*x(k+1)+B*u(k)=0 
               Zeros(1:N(j),1:2*N(j)), (Hukp1-Huk), blkdiag(vx(j)*T,ds*Eye(1:N(j)-1,1:N(j)-1))]; % u'(k)*ds = u(k+1) - u(k))
               
    beq_car = [(-A*xk(:,j)); Zeros(1:(N(j)-1)*2,1); uk(j); Zeros(1:(N(j)-1),1)];
    
    Aeq = blkdiag(Aeq,Aeq_car);
    beq = [beq;beq_car];

      
% % Inequality Constraints
 
    Ain_car = [kron(Eye(1:N(j),1:N(j)),C'), Zeros(1:N(j),1:2*N(j));  % 1/vx >= 1/vmax                   1)
               kron(Eye(1:N(j),1:N(j)),-C'), Zeros(1:N(j),1:2*N(j)); % -1/vx >= -1/vmin                 2)
               kron(Eye(1:N(j),1:N(j)),3*amax*vx(j)^2*C'), Eye(1:N(j),1:N(j)), Zeros(1:N(j),1:N(j));  % u >= umin     3)
               kron(Eye(1:N(j),1:N(j)),-3*amin*vx(j)^2*C'), -Eye(1:N(j),1:N(j)), Zeros(1:N(j),1:N(j))]; % -u >= -umax 4)
           
    bin_car = [Ones(1:N(j),1).*1/vmax;             % 1)
               Ones(1:N(j),1).*(-1/vmin);          % 2)
               Ones(1:N(j),1).*(2*amax/vx(j)^3);   % 3)
               Ones(1:N(j),1).*(-2*amin/vx(j)^3)];  % 4)
    
    Ain = blkdiag(Ain,Ain_car);
    bin = [bin;bin_car];
     
    end
end


% % Cronologic crossing order Car 1-> Car 2 -> Car 3
% % -------------------

% % index for cars inside control region
ind = find(dist2Int< contR &  dist2Int > -(contR+critZ));
leni = length(ind); % number of cars inside the crontrol region

ns = 0; % number of added slack variables

if  leni >= 2 % if 2 or more cars is in the control region

    for j=1: length(ind)-1 % itterate all vehicle pairs
        leave = (dist2Int(ind(j))+critZ); % index [m] for first car to leave
        enter = (dist2Int(ind(j+1))); % index [m] for next car to enter
        
        % if the indexes is positive add a slack variable for the vehicle pair
        if min(leave,enter) >= 1 
            ns = ns+1;

            Ain = blkdiag(Ain,zeros(3,1)); % Add three rows for slack constraint
            bin = vertcat(bin,zeros(3,1)); % -||-
            
            Ain(end-2,2*leave-1 + 4*sum(N(1:(ind(j)-1)))) = -1;  % 1)
            Ain(end-2,2*enter-1 + 4*sum(N(1:(ind(j+1)-1)))) = 1; % 1)
            
            Ain(end-1,2*leave-1 + 4*sum(N(1:(ind(j)-1)))) = -1;  % 2)
            Ain(end-1,2*enter-1 + 4*sum(N(1:(ind(j+1)-1)))) = 1; % 2)
            Ain(end-1,end) = 1;                                  % 2)
            bin(end-1) = tdiff;
            
            Ain(end,end) = 1;                                    % 3)
            
            % 1) t(car_2(enter)) - t(car_1(leave)) >= 0
            % 2) t(car_2(enter)) - t(car_1(leave)) + q >= tdiff
            % 3) q >= 0  
    
        end
    end
end
% 
if ns > 0
    Aeq = [Aeq, Zeros(1:size(Aeq,1),1:ns)]; % Add variable q for each slack variable
    Hm = blkdiag(Hm,kron(Eye(1:ns,1:ns),2*w(4)));
    f = [f; Zeros(1:ns,1)];
end

% % If any car is within the control region the MPC will optimize the path
% % for all cars within the controlling region.
if ~isempty(Hm)
    
   
    [L,~] = chol(Hm,'lower');
    Linv = inv(L);
    x = zeros(size(Linv,2),1);
    opt= mpcqpsolverOptions('double');
    
   % tic;
    [x,exflag] = mpcqpsolver(Linv,f,Ain,bin,Aeq,beq,false(size(bin)),opt); %,options);
    % time = toc;
    
    if exflag == -2
        disp('Error: exflag == 2 ');
    end
    
    for j=1:numCars
        
        prev = 4*sum(N(1:j-1));
        
        if N(j) > 1
            longAcc(j) = -x(2*N(j)+1 + prev)/ x(2 + prev)^3;
        else
            longAcc(j) = 0; 
        end
        
    end
    
else
    for j=1:numCars
        longAcc(j) = 0;
    end
end
end
